simulink model "forwardConverter"  (R2019a)
settings: Solver=VariableStepAuto  StartTime=0  StopTime=0.1  MaxStep=1e-4  RelTol=1e-4  EnableMultiTasking=on
libraries: powerlib x22, powerlib_meascontrol x4, simulink x2
Description:
  | Copyright 2008-2019 The MathWorks, Inc.
settings Model: Creator=MathWorks  LastModifiedBy=Burak
settings SolverCC: SolverResetMethod=Robust
settings OptimizationCC: LifeSpan=inf
settings DebuggingCC: ReadBeforeWriteMsg=DisableAll  WriteAfterWriteMsg=DisableAll  WriteAfterReadMsg=DisableAll  MultiTaskDSMMsg=none  SFUnexpectedBacktrackingDiag=warning  SFNoUnconditionalDefaultTransitionDiag=warning  SFExecutionAtInitializationDiag=none  ArithmeticOperatorsInVariantConditions=warning
settings ModelReferenceCC: UpdateModelReferenceTargets=IfOutOfDate
settings SFSimCC: SFSimEcho=off  SimUseLocalCustomCode=off
settings RTWCC: RTWUseLocalCustomCode=off
settings CodeAppCC: StateflowObjectComments=on
settings GRTTargetCC: TargetLangStandard=C89/C90 (ANSI)  GeneratePreprocessorConditionals=Disable all
settings ConfigComp: CovMetricSettings=dw  CovHtmlReporting=on  CovSaveCumulativeToWorkspaceVar=on  CovSaveSingleToWorkspaceVar=on  CovExternalEMLEnable=off
settings SimscapeCC: SimscapeNormalizeSystem=off  SimscapeNominalValues={1, 'bar'; 1, 'cm^3/s'; 1, 'bar*kg/s'; 1, 'kJ/kg'; 1, 'kW'; }

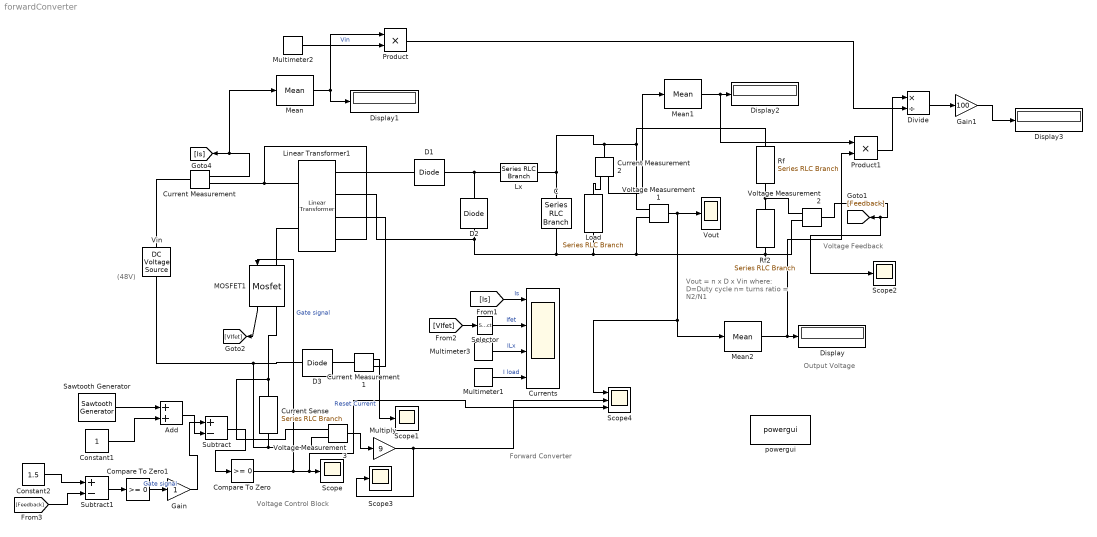
== system forwardConverter ==
  note: Vout = n x D x Vin
      | where: D=Duty cycle
      | n= turns ratio = N2/N1
  note: (48V)
  note: Forward Converter
  note: Output Voltage
  note: Voltage Control Block
  note: Voltage Feedback
  Add : Sum
  C : powerlib/Elements/Series RLC Branch  LConnTagsString=__new0  RConnTagsString=__new0  BranchType=C  Resistance=1e-4  Inductance=200e-6  SetiL0=off  InitialCurrent=0  Capacitance=1e-3  Setx0=off  InitialVoltage=0  Measurements=None
      settings: SourceProductName=Simscape Electrical
  Compare To Zero : simulink/Logic and Bit Operations/Compare To Zero  relop=>=  OutDataTypeStr=boolean
  Compare To Zero1 : simulink/Logic and Bit Operations/Compare To Zero  relop=>=  OutDataTypeStr=boolean
  Constant1 : Constant
  Constant2 : Constant  Value=1.5
  Current Measurement : powerlib/Measurements/Current Measurement  PhasorSimulation=off  OutputType=Complex  PSBequivalent=0
      settings: SourceProductName=Simscape Electrical
  Current Measurement1 : powerlib/Measurements/Current Measurement  PhasorSimulation=off  OutputType=Complex  PSBequivalent=0
      settings: SourceProductName=Simscape Electrical
  Current Measurement2 : powerlib/Measurements/Current Measurement  PhasorSimulation=off  OutputType=Complex  PSBequivalent=0
      settings: SourceProductName=Simscape Electrical
  Current Sense : powerlib/Elements/Series RLC Branch  LConnTagsString=__new0  RConnTagsString=__new0  BranchType=R  Resistance=0.01  Inductance=200e-6  SetiL0=off  InitialCurrent=0  Capacitance=400e-6  Setx0=off  InitialVoltage=0  Measurements=Branch current
      settings: SourceProductName=Simscape Electrical
  Currents : Scope  NumInputPorts=4
  D1 : powerlib/Power Electronics/Diode  Ron=1e-3  Lon=0  Vf=1  IC=0  UseSnubber=off  Rs=inf  Cs=0  Measurements=off
      settings: SourceProductName=Simscape Electrical
  D2 : powerlib/Power Electronics/Diode  Ron=1e-3  Lon=0  Vf=1  IC=0  UseSnubber=off  Rs=inf  Cs=0  Measurements=off
      settings: SourceProductName=Simscape Electrical
  D3 : powerlib/Power Electronics/Diode  Ron=1e-3  Lon=0  Vf=1  IC=0  UseSnubber=off  Rs=inf  Cs=0  Measurements=off
      settings: SourceProductName=Simscape Electrical
  Display{,1..3} (4 alike) : Display
  Divide : Product  Inputs=*/
  Gain : Gain
  Gain1 : Gain  Gain=100
  Linear Transformer1 : powerlib/Elements/Linear Transformer  UNITS=SI  NominalPower=[ 250e6 100000 ]  winding1=[48 0 0]  winding2=[96 0 0]  ThreeWindings=on  winding3=[48 0 0]  RmLm=[5e3 12e-3]  Measurements=None  DataType=on
      settings: SourceProductName=Simscape Electrical
  Load : powerlib/Elements/Series RLC Branch  LConnTagsString=__new0  RConnTagsString=__new0  BranchType=R  Resistance=6  Inductance=200e-6  SetiL0=off  InitialCurrent=0  Capacitance=400e-6  Setx0=off  InitialVoltage=0  Measurements=Branch current
      settings: SourceProductName=Simscape Electrical
  Lx : powerlib/Elements/Series RLC Branch  LConnTagsString=__new0  RConnTagsString=__new0  BranchType=L  Resistance=10  Inductance=4e-3  SetiL0=off  InitialCurrent=0  Capacitance=400e-6  Setx0=off  InitialVoltage=0  Measurements=Branch current
      settings: SourceProductName=Simscape Electrical
  MOSFET1 : powerlib/Power Electronics/Mosfet  Ron=1e-3  Lon=0  Rd=1e-3  Vfd=0  IC=0  Rs=1e6  Cs=inf  Measurements=on
      settings: SourceProductName=Simscape Electrical
  Mean : powerlib_meascontrol/Measurements/Mean  Freq=60  Vinit=0  Ts=0
      settings: SourceProductName=Simscape Electrical
  Mean1 : powerlib_meascontrol/Measurements/Mean  Freq=60  Vinit=0  Ts=0
      settings: SourceProductName=Simscape Electrical
  Mean2 : powerlib_meascontrol/Measurements/Mean  Freq=60  Vinit=0  Ts=0
      settings: SourceProductName=Simscape Electrical
  Multimeter1 : powerlib/Measurements/Multimeter  PhasorSimulation=off  OutputType=Complex  sel=3  L=6  Gain=1  yselected={'Ib: Load'};  PSBOutputType=1  PSBequivalent=0  AxesSetting=[0,0.1,-100,100]  Display=0  SavedBlockNames=-11
      settings: SourceProductName=Simscape Electrical
  Multimeter2 : powerlib/Measurements/Multimeter  PhasorSimulation=off  OutputType=Complex  sel=1  L=6  Gain=1  yselected={'Usrc: Vin'};  PSBOutputType=1  PSBequivalent=0  AxesSetting=[0,0.1,-100,100]  Display=0  SavedBlockNames=-11
      settings: SourceProductName=Simscape Electrical
  Multimeter3 : powerlib/Measurements/Multimeter  PhasorSimulation=off  OutputType=Complex  sel=4  L=6  Gain=1  yselected={'Ib: Lx'};  PSBOutputType=1  PSBequivalent=0  AxesSetting=[0,0.1,-100,100]  Display=0  SavedBlockNames=-11
      settings: SourceProductName=Simscape Electrical
  Multiply : Gain  Gain=9
  Product : Product
  Product1 : Product
  Rf : powerlib/Elements/Series RLC Branch  LConnTagsString=__new0  RConnTagsString=__new0  BranchType=R  Resistance=9e6  Inductance=200e-6  SetiL0=off  InitialCurrent=0  Capacitance=400e-6  Setx0=off  InitialVoltage=0  Measurements=Branch current
      settings: SourceProductName=Simscape Electrical
  Rf2 : powerlib/Elements/Series RLC Branch  LConnTagsString=__new0  RConnTagsString=__new0  BranchType=R  Resistance=1e6  Inductance=200e-6  SetiL0=off  InitialCurrent=0  Capacitance=400e-6  Setx0=off  InitialVoltage=0  Measurements=Branch current
      settings: SourceProductName=Simscape Electrical
  Sawtooth Generator : powerlib_meascontrol/Pulse & Signal Generators/Sawtooth Generator  Freq=100000  Phase=180  Ts=0
      settings: SourceProductName=Simscape Electrical
  Scope{,1..3} (4 alike) : Scope
  Scope4 : Scope  NumInputPorts=3
  Selector : Selector  InputPortWidth=2  IndexOptions=Index vector (dialog)  Indices=1  OutputSizes=1
  Subtract : Sum  Inputs=+-
  Subtract1 : Sum  Inputs=+-
  Vin : powerlib/Electrical Sources/DC Voltage Source  Amplitude=48  Measurements=Voltage
      settings: SourceProductName=Simscape Electrical
  Voltage Measurement1 : powerlib/Measurements/Voltage Measurement  PhasorSimulation=off  OutputType=Complex  PSBequivalent=0
      settings: SourceProductName=Simscape Electrical
  Voltage Measurement2 : powerlib/Measurements/Voltage Measurement  PhasorSimulation=off  OutputType=Complex  PSBequivalent=0
      settings: SourceProductName=Simscape Electrical
  Voltage Measurement3 : powerlib/Measurements/Voltage Measurement  PhasorSimulation=off  OutputType=Complex  PSBequivalent=0
      settings: SourceProductName=Simscape Electrical
  Vout : Scope
  powergui : powerlib/powergui  Priority=1  SimulationMode=Continuous  SampleTime=50e-6  frequency=60  Iterations=50  frequencyindice=0  Pbase=100e6  ErrMax=1e-4  UnitsV=kV  UnitsW=MW  buscounter=0  FunctionMessages=off  echomessages=off  EnableUseOfTLC=off  CurrentSourceSwitches=off  DisableSnubberDevices=off  DisableRonSwitches=off  DisableVfSwitches=off  DisplayEquations=off  AutomaticDiscreteSolvers=off  SolverType=Tustin/Backward Euler (TBE)  Interpol=off  ExternalGateDelay=off  methode=off  Ts=100  x0status=blocks  SPID=on  SwTol=0  HookPort=off  NonlinearTolerance=0  nMaxIteration=15  ContinueOnMaxIteration=off  RestoreLinks=warning  ResistiveCurrentMeasurement=off  Frange=[0:2:500]  Ylog=off  Xlog=on  ShowGrid=off  save=off  variable=ZData  structure=0  ZoomFFT=off  StartTime=0.0  cycles=1  DisplayStyle=1  fundamental=60  FreqAxis=off  MaxFrequency=1000  frequencyindicesteady=1  RmsSteady=1  display=off
      settings: SourceProductName=Simscape Electrical
  wires:
  Compare To Zero/1 -> MOSFET1/1, Scope4/3, Scope/1  "Gate signal"
  Voltage Measurement1/1 -> Mean2/1, Scope4/1, Vout/1
  MOSFET1/1 -> [VIfet]
  [VIfet] -> Selector/1
  [Is] -> Currents/1  "Is"
  Multimeter3/1 -> Currents/3  "ILx"
  Multimeter1/1 -> Currents/4  "I load"
  Selector/1 -> Currents/2  "Ifet"
  Mean2/1 -> Product1/2, Display/1
  Voltage Measurement2/1 -> Scope2/1, [Feedback]
  Subtract/1 -> Compare To Zero/1
  Constant1/1 -> Add/2
  Sawtooth Generator/1 -> Add/1
  Current Measurement1/1 -> Scope1/1  "Reset Current"
  Add/1 -> Subtract/2
  Constant2/1 -> Subtract1/1
  [Feedback] -> Subtract1/2
  Subtract1/1 -> Compare To Zero1/1
  Compare To Zero1/1 -> Gain/1  "Gate signal"
  Gain/1 -> Subtract/1
  Voltage Measurement3/1 -> Multiply/1
  Multiply/1 -> Scope4/2, Scope3/1
  Current Measurement/1 -> Mean/1, [Is]
  Current Measurement2/1 -> Mean1/1
  Mean1/1 -> Product1/1, Display2/1
  Mean/1 -> Product/1, Display1/1
  Multimeter2/1 -> Product/2  "Vin"
  Product/1 -> Divide/2
  Product1/1 -> Divide/1
  Divide/1 -> Gain1/1
  Gain1/1 -> Display3/1
  connections:
  Lx/RConn1 -- Current Measurement2/LConn1 -- Voltage Measurement1/LConn1 -- Rf/LConn1 -- C/LConn1
  D2/LConn1 -- C/RConn1 -- Voltage Measurement2/LConn2 -- Rf2/RConn1 -- Voltage Measurement1/LConn2 -- Load/RConn1 -- Linear Transformer1/RConn2
  Linear Transformer1/LConn2 -- MOSFET1/LConn1
  Vin/LConn1 -- Voltage Measurement3/LConn2 -- Current Sense/RConn1 -- D3/LConn1
  Current Measurement/RConn1 -- Linear Transformer1/RConn4 -- Linear Transformer1/LConn1
  Linear Transformer1/RConn1 -- D1/LConn1
  D2/RConn1 -- D1/RConn1 -- Lx/LConn1
  Vin/RConn1 -- Current Measurement/LConn1
  Rf/RConn1 -- Voltage Measurement2/LConn1 -- Rf2/LConn1
  Current Measurement1/LConn1 -- D3/RConn1
  Linear Transformer1/RConn3 -- Current Measurement1/RConn1
  MOSFET1/RConn1 -- Voltage Measurement3/LConn1 -- Current Sense/LConn1
  Load/LConn1 -- Current Measurement2/RConn1
